simulink model "TVModel_Simulation"  (R2022a)
settings: Solver=FixedStepDiscrete  StartTime=0.0  StopTime=200  FixedStep=0.02  MaxStep=0.01  RelTol=1e-3
undefined symbols (not defined in the file or in its folder): TV
libraries: simulink x5, simulink_extras x3, dspstat3 x2, sharedTrackingLibrary x1, slpidlib x1, eeGeneralControl x1
(part 4 of 4)

== matlab function TVModel_Simulation/Subsystem/Subsystem1/Torque Distribution/MPC/ States/Extended Kalman Filter/state_update_kalman_simulink/f(x,u) ==
  data: x input; u input; xout output
function xout = state_update_kalman_simulink(x,u)

%% ~~~~~~~~~~~~~~~~~~~~~~~~~~~~~ Intro ~~~~~~~~~~~~~~~~~~~~~~~~~~~~~~~~~~~~
dt = 1/50;
%% ~~~~~~~~~~~~~~~~~~~~~~~~ Car parameters ~~~~~~~~~~~~~~~~~~~~~~~~~~~~~~~~
xout = zeros(3,1);
% ~~~~~~~~~~~~~~~~~~~~~~~~ General Parameters ~~~~~~~~~~~~~~~~~~~~~~~~~~~~~
g   = 9.81;            % [m/s^2]                          
wd  = 0.5;             % [~]         
wb  = 1.53;            % [~]          
tf  = 1.27;            % [m]          
tr  = 1.27;            % [m]          
m   = 195+75;          % [Kg]            
Iz  = 120;             % [Kg*m^2]         
a   = wb*wd;           % [m]            
b   = wb - a;          % [m]            
hcog = 0.29;           % [m]           
Fzf  = m*g/2*(wd);     % [N]                 
Fzr  = m*g/2*(1-wd);   % [N]                   
tau = 13.5;            % [~]          
rs  = 0.235;           % [m]           

% ~~~~~~~~~~~~~~~~~~~~~~~~~~~ Aero parameters ~~~~~~~~~~~~~~~~~~~~~~~~~~~~~
wbaero = 0.5542;       % [~]           
hcop = 0.576;          % [m]      
rho = 1.225;           % [Kg/m^3]     
CdA = 1.708;           % [m]     
ClA = 5.14;            % [m]    

% ~~~~~~~~~~~~~~~~~~~~~~~~~~ Other parameters ~~~~~~~~~~~~~~~~~~~~~~~~~~~~~

% ~~~~~~~~~~~~~~~~~~~~~~~~~~~ Set up states  ~~~~~~~~~~~~~~~~~~~~~~~~~~~~~~
vx = x(1);
vy = x(2);
r  = x(3);

% ~~~~~~~~~~~~~~~~~~~~~~~~~~~ Set up parameters ~~~~~~~~~~~~~~~~~~~~~~~~~~~
% delta    = u(1);
% kappa_FL = u(2);
% kappa_FR = u(3);
% kappa_RL = u(4);
% kappa_RR = u(5);
% Tbrk_FL  = u(6);
% Tbrk_FR  = u(7);
% Tbrk_RL  = u(8);
% Tbrk_RR  = u(9);
% ay       = u(10);
% ax       = u(11);
% T_FL     = u(12);
% T_FR     = u(13);
% T_RL     = u(14);
% T_RR     = u(15);

delta    = u(1);
kappa_FL = u(2);
kappa_FR = u(3);
kappa_RL = u(4);
kappa_RR = u(5);
T_FL     = u(6);
T_FR     = u(7);
T_RL     = u(8);
T_RR     = u(9);

ax = 0; ay = 0;
Tbrk_FL  = 0;
Tbrk_FR  = 0;
Tbrk_RL  = 0;
Tbrk_RR  = 0;
%% ~~~~~~~~~~~~~~~~~~~~~~~~~~ System Dynamics ~~~~~~~~~~~~~~~~~~~~~~~~~~~~~~

% ~~~~~~~~~~~~~~~~~~~~~~~~~~~ Aerodynamics ~~~~~~~~~~~~~~~~~~~~~~~~~~~~~~~~
Faerox = 0.5*rho*CdA*vx^2;
Faeroz = 0.5*rho*ClA*vx^2;

% ~~~~~~~~~~~~~~~~~~~~~~~~~~~ Slip Angles ~~~~~~~~~~~~~~~~~~~~~~~~~~~~~~~~~
alpha_FL =  (((vy + r*a)./(vx - r*tf/2)) - delta);
alpha_FR =  (((vy + r*a)./(vx + r*tf/2)) - delta);
alpha_RL =  (((vy - r*b)./(vx - r*tr/2)));     
alpha_RR =  (((vy - r*b)./(vx + r*tr/2)));     

% ~~~~~~~~~~~~~~~~~~~~~~~~~~~ Vertical loads ~~~~~~~~~~~~~~~~~~~~~~~~~~~~~~
Fz_FL = Fzf - 0.5*(m/tf*hcog).*ay + 0.5*Faeroz*wbaero - 0.5*Faerox/wb*hcop - 0.5*(m/wb*hcog).*ax;
Fz_FR = Fzf + 0.5*(m/tf*hcog).*ay + 0.5*Faeroz*wbaero - 0.5*Faerox/wb*hcop - 0.5*(m/wb*hcog).*ax;
Fz_RL = Fzr - 0.5*(m/tr*hcog).*ay + 0.5*Faeroz*(1-wbaero) + 0.5*Faerox/wb*hcop + 0.5*(m/wb*hcog).*ax;
Fz_RR = Fzr + 0.5*(m/tr*hcog).*ay + 0.5*Faeroz*(1-wbaero) + 0.5*Faerox/wb*hcop + 0.5*(m/wb*hcog).*ax;

% ~~~~~~~~~~~~~~~~~~~~~~~~~~ Lateral forces ~~~~~~~~~~~~~~~~~~~~~~~~~~~~~~~
muY = 1.5;
Fy_FL = (cos(0.95064*atan((41.4696*(kappa_FL - 0.00000078224999999999995925481499625675*Fz_FL + 0.00056678999999999995877686398415563))/((13.456699999999999661781657778192*alpha_FL - 0.51027806399999998717476046294905)^2 + 1.0)^(1/2) + (0.0012906*Fz_FL - 2.3215)*(atan((41.4696*(kappa_FL - 0.00000078224999999999995925481499625675*Fz_FL + 0.00056678999999999995877686398415563))/((13.456699999999999661781657778192*alpha_FL - 0.51027806399999998717476046294905)^2 + 1.0)^(1/2)) - (41.4696*(kappa_FL - 0.00000078224999999999995925481499625675*Fz_FL + 0.00056678999999999995877686398415563))/((13.456699999999999661781657778192*alpha_FL - 0.51027806399999998717476046294905)^2 + 1.0)^(1/2))))*(0.93*Fz_FL*(0.000071017999999999997795541162304289*Fz_FL - 0.14887799999999999779554116230429) - 0.93*Fz_FL*(0.00074656*Fz_FL + 0.37814) + Fz_FL*muY*sin(1.1962*atan((28888.097815192522084544179961085*sin(2.0*atan(0.00077863498204218704389788477193347*Fz_FL))*(0.000001140900000000000030428437547414*Fz_FL - 1.0*alpha_FL + (0.93*Fz_FL*(0.00074656*Fz_FL + 0.37814) + 1.1538900000000000822808488010196*Fz_FL*(0.00023917*Fz_FL - 1.57477))/(28888.097815192522084544179961085*sin(2.0*atan(0.00077863498204218704389788477193347*Fz_FL)) - 0.01) + 0.0023905000000000000467265115489113))/(1.1962*Fz_FL*muY + 0.01) - 1.0*(atan((28888.097815192522084544179961085*sin(2.0*atan(0.00077863498204218704389788477193347*Fz_FL))*(0.000001140900000000000030428437547414*Fz_FL - 1.0*alpha_FL + (0.93*Fz_FL*(0.00074656*Fz_FL + 0.37814) + 1.1538900000000000822808488010196*Fz_FL*(0.00023917*Fz_FL - 1.57477))/(28888.097815192522084544179961085*sin(2.0*atan(0.00077863498204218704389788477193347*Fz_FL)) - 0.01) + 0.0023905000000000000467265115489113))/(1.1962*Fz_FL*muY + 0.01)) - (28888.097815192522084544179961085*sin(2.0*atan(0.00077863498204218704389788477193347*Fz_FL))*(0.000001140900000000000030428437547414*Fz_FL - 1.0*alpha_FL + (0.93*Fz_FL*(0.00074656*Fz_FL + 0.37814) + 1.1538900000000000822808488010196*Fz_FL*(0.00023917*Fz_FL - 1.57477))/(28888.097815192522084544179961085*sin(2.0*atan(0.00077863498204218704389788477193347*Fz_FL)) - 0.01) + 0.0023905000000000000467265115489113))/(1.1962*Fz_FL*muY + 0.01))*(0.000039933999999999997276844965199416*Fz_FL - 0.52068399999999999727684496519942)*(0.47036*sign(0.000001140900000000000030428437547414*Fz_FL - 1.0*alpha_FL + (0.93*Fz_FL*(0.00074656*Fz_FL + 0.37814) + 1.1538900000000000822808488010196*Fz_FL*(0.00023917*Fz_FL - 1.57477))/(28888.097815192522084544179961085*sin(2.0*atan(0.00077863498204218704389788477193347*Fz_FL)) - 0.01) + 0.0023905000000000000467265115489113) - 7.9286)))))/cos(0.95064*atan((41.4696*(0.00000078224999999999995925481499625675*Fz_FL - 0.00056678999999999995877686398415563))/((13.456699999999999661781657778192*alpha_FL - 0.51027806399999998717476046294905)^2 + 1.0)^(1/2) + (0.0012906*Fz_FL - 2.3215)*(atan((41.4696*(0.00000078224999999999995925481499625675*Fz_FL - 0.00056678999999999995877686398415563))/((13.456699999999999661781657778192*alpha_FL - 0.51027806399999998717476046294905)^2 + 1.0)^(1/2)) - (41.4696*(0.00000078224999999999995925481499625675*Fz_FL - 0.00056678999999999995877686398415563))/((13.456699999999999661781657778192*alpha_FL - 0.51027806399999998717476046294905)^2 + 1.0)^(1/2)))) - (1.0*Fz_FL*muY*sin(1.9085*atan(16.5046*kappa_FL))*(0.0000027179999999999999299449271461526*Fz_FL - 1.1553830000000000000737188088351))/(225.17103248999997449603881705116*alpha_FL^2 + 1.0)^(1/2) + 400;
Fy_FR = (cos(0.95064*atan((41.4696*(kappa_FR - 0.00000078224999999999995925481499625675*Fz_FR + 0.00056678999999999995877686398415563))/((13.456699999999999661781657778192*alpha_FR - 0.51027806399999998717476046294905)^2 + 1.0)^(1/2) + (0.0012906*Fz_FR - 2.3215)*(atan((41.4696*(kappa_FR - 0.00000078224999999999995925481499625675*Fz_FR + 0.00056678999999999995877686398415563))/((13.456699999999999661781657778192*alpha_FR - 0.51027806399999998717476046294905)^2 + 1.0)^(1/2)) - (41.4696*(kappa_FR - 0.00000078224999999999995925481499625675*Fz_FR + 0.00056678999999999995877686398415563))/((13.456699999999999661781657778192*alpha_FR - 0.51027806399999998717476046294905)^2 + 1.0)^(1/2))))*(0.93*Fz_FR*(0.000071017999999999997795541162304289*Fz_FR - 0.14887799999999999779554116230429) - 0.93*Fz_FR*(0.00074656*Fz_FR + 0.37814) + Fz_FR*muY*sin(1.1962*atan((28888.097815192522084544179961085*sin(2.0*atan(0.00077863498204218704389788477193347*Fz_FR))*(0.000001140900000000000030428437547414*Fz_FR - 1.0*alpha_FR + (0.93*Fz_FR*(0.00074656*Fz_FR + 0.37814) + 1.1538900000000000822808488010196*Fz_FR*(0.00023917*Fz_FR - 1.57477))/(28888.097815192522084544179961085*sin(2.0*atan(0.00077863498204218704389788477193347*Fz_FR)) - 0.01) + 0.0023905000000000000467265115489113))/(1.1962*Fz_FR*muY + 0.01) - 1.0*(atan((28888.097815192522084544179961085*sin(2.0*atan(0.00077863498204218704389788477193347*Fz_FR))*(0.000001140900000000000030428437547414*Fz_FR - 1.0*alpha_FR + (0.93*Fz_FR*(0.00074656*Fz_FR + 0.37814) + 1.1538900000000000822808488010196*Fz_FR*(0.00023917*Fz_FR - 1.57477))/(28888.097815192522084544179961085*sin(2.0*atan(0.00077863498204218704389788477193347*Fz_FR)) - 0.01) + 0.0023905000000000000467265115489113))/(1.1962*Fz_FR*muY + 0.01)) - (28888.097815192522084544179961085*sin(2.0*atan(0.00077863498204218704389788477193347*Fz_FR))*(0.000001140900000000000030428437547414*Fz_FR - 1.0*alpha_FR + (0.93*Fz_FR*(0.00074656*Fz_FR + 0.37814) + 1.1538900000000000822808488010196*Fz_FR*(0.00023917*Fz_FR - 1.57477))/(28888.097815192522084544179961085*sin(2.0*atan(0.00077863498204218704389788477193347*Fz_FR)) - 0.01) + 0.0023905000000000000467265115489113))/(1.1962*Fz_FR*muY + 0.01))*(0.000039933999999999997276844965199416*Fz_FR - 0.52068399999999999727684496519942)*(0.47036*sign(0.000001140900000000000030428437547414*Fz_FR - 1.0*alpha_FR + (0.93*Fz_FR*(0.00074656*Fz_FR + 0.37814) + 1.1538900000000000822808488010196*Fz_FR*(0.00023917*Fz_FR - 1.57477))/(28888.097815192522084544179961085*sin(2.0*atan(0.00077863498204218704389788477193347*Fz_FR)) - 0.01) + 0.0023905000000000000467265115489113) - 7.9286)))))/cos(0.95064*atan((41.4696*(0.00000078224999999999995925481499625675*Fz_FR - 0.00056678999999999995877686398415563))/((13.456699999999999661781657778192*alpha_FR - 0.51027806399999998717476046294905)^2 + 1.0)^(1/2) + (0.0012906*Fz_FR - 2.3215)*(atan((41.4696*(0.00000078224999999999995925481499625675*Fz_FR - 0.00056678999999999995877686398415563))/((13.456699999999999661781657778192*alpha_FR - 0.51027806399999998717476046294905)^2 + 1.0)^(1/2)) - (41.4696*(0.00000078224999999999995925481499625675*Fz_FR - 0.00056678999999999995877686398415563))/((13.456699999999999661781657778192*alpha_FR - 0.51027806399999998717476046294905)^2 + 1.0)^(1/2)))) - (1.0*Fz_FR*muY*sin(1.9085*atan(16.5046*kappa_FR))*(0.0000027179999999999999299449271461526*Fz_FR - 1.1553830000000000000737188088351))/(225.17103248999997449603881705116*alpha_FR^2 + 1.0)^(1/2) + 400;
Fy_RL = (cos(0.95064*atan((41.4696*(kappa_RL - 0.00000078224999999999995925481499625675*Fz_RL + 0.00056678999999999995877686398415563))/((13.456699999999999661781657778192*alpha_RL - 0.51027806399999998717476046294905)^2 + 1.0)^(1/2) + (0.0012906*Fz_RL - 2.3215)*(atan((41.4696*(kappa_RL - 0.00000078224999999999995925481499625675*Fz_RL + 0.00056678999999999995877686398415563))/((13.456699999999999661781657778192*alpha_RL - 0.51027806399999998717476046294905)^2 + 1.0)^(1/2)) - (41.4696*(kappa_RL - 0.00000078224999999999995925481499625675*Fz_RL + 0.00056678999999999995877686398415563))/((13.456699999999999661781657778192*alpha_RL - 0.51027806399999998717476046294905)^2 + 1.0)^(1/2))))*(0.93*Fz_RL*(0.000071017999999999997795541162304289*Fz_RL - 0.14887799999999999779554116230429) - 0.93*Fz_RL*(0.00074656*Fz_RL + 0.37814) + Fz_RL*muY*sin(1.1962*atan((28888.097815192522084544179961085*sin(2.0*atan(0.00077863498204218704389788477193347*Fz_RL))*(0.000001140900000000000030428437547414*Fz_RL - 1.0*alpha_RL + (0.93*Fz_RL*(0.00074656*Fz_RL + 0.37814) + 1.1538900000000000822808488010196*Fz_RL*(0.00023917*Fz_RL - 1.57477))/(28888.097815192522084544179961085*sin(2.0*atan(0.00077863498204218704389788477193347*Fz_RL)) - 0.01) + 0.0023905000000000000467265115489113))/(1.1962*Fz_RL*muY + 0.01) - 1.0*(atan((28888.097815192522084544179961085*sin(2.0*atan(0.00077863498204218704389788477193347*Fz_RL))*(0.000001140900000000000030428437547414*Fz_RL - 1.0*alpha_RL + (0.93*Fz_RL*(0.00074656*Fz_RL + 0.37814) + 1.1538900000000000822808488010196*Fz_RL*(0.00023917*Fz_RL - 1.57477))/(28888.097815192522084544179961085*sin(2.0*atan(0.00077863498204218704389788477193347*Fz_RL)) - 0.01) + 0.0023905000000000000467265115489113))/(1.1962*Fz_RL*muY + 0.01)) - (28888.097815192522084544179961085*sin(2.0*atan(0.00077863498204218704389788477193347*Fz_RL))*(0.000001140900000000000030428437547414*Fz_RL - 1.0*alpha_RL + (0.93*Fz_RL*(0.00074656*Fz_RL + 0.37814) + 1.1538900000000000822808488010196*Fz_RL*(0.00023917*Fz_RL - 1.57477))/(28888.097815192522084544179961085*sin(2.0*atan(0.00077863498204218704389788477193347*Fz_RL)) - 0.01) + 0.0023905000000000000467265115489113))/(1.1962*Fz_RL*muY + 0.01))*(0.000039933999999999997276844965199416*Fz_RL - 0.52068399999999999727684496519942)*(0.47036*sign(0.000001140900000000000030428437547414*Fz_RL - 1.0*alpha_RL + (0.93*Fz_RL*(0.00074656*Fz_RL + 0.37814) + 1.1538900000000000822808488010196*Fz_RL*(0.00023917*Fz_RL - 1.57477))/(28888.097815192522084544179961085*sin(2.0*atan(0.00077863498204218704389788477193347*Fz_RL)) - 0.01) + 0.0023905000000000000467265115489113) - 7.9286)))))/cos(0.95064*atan((41.4696*(0.00000078224999999999995925481499625675*Fz_RL - 0.00056678999999999995877686398415563))/((13.456699999999999661781657778192*alpha_RL - 0.51027806399999998717476046294905)^2 + 1.0)^(1/2) + (0.0012906*Fz_RL - 2.3215)*(atan((41.4696*(0.00000078224999999999995925481499625675*Fz_RL - 0.00056678999999999995877686398415563))/((13.456699999999999661781657778192*alpha_RL - 0.51027806399999998717476046294905)^2 + 1.0)^(1/2)) - (41.4696*(0.00000078224999999999995925481499625675*Fz_RL - 0.00056678999999999995877686398415563))/((13.456699999999999661781657778192*alpha_RL - 0.51027806399999998717476046294905)^2 + 1.0)^(1/2)))) - (1.0*Fz_RL*muY*sin(1.9085*atan(16.5046*kappa_RL))*(0.0000027179999999999999299449271461526*Fz_RL - 1.1553830000000000000737188088351))/(225.17103248999997449603881705116*alpha_RL^2 + 1.0)^(1/2) + 400;
Fy_RR = (cos(0.95064*atan((41.4696*(kappa_RR - 0.00000078224999999999995925481499625675*Fz_RR + 0.00056678999999999995877686398415563))/((13.456699999999999661781657778192*alpha_RR - 0.51027806399999998717476046294905)^2 + 1.0)^(1/2) + (0.0012906*Fz_RR - 2.3215)*(atan((41.4696*(kappa_RR - 0.00000078224999999999995925481499625675*Fz_RR + 0.00056678999999999995877686398415563))/((13.456699999999999661781657778192*alpha_RR - 0.51027806399999998717476046294905)^2 + 1.0)^(1/2)) - (41.4696*(kappa_RR - 0.00000078224999999999995925481499625675*Fz_RR + 0.00056678999999999995877686398415563))/((13.456699999999999661781657778192*alpha_RR - 0.51027806399999998717476046294905)^2 + 1.0)^(1/2))))*(0.93*Fz_RR*(0.000071017999999999997795541162304289*Fz_RR - 0.14887799999999999779554116230429) - 0.93*Fz_RR*(0.00074656*Fz_RR + 0.37814) + Fz_RR*muY*sin(1.1962*atan((28888.097815192522084544179961085*sin(2.0*atan(0.00077863498204218704389788477193347*Fz_RR))*(0.000001140900000000000030428437547414*Fz_RR - 1.0*alpha_RR + (0.93*Fz_RR*(0.00074656*Fz_RR + 0.37814) + 1.1538900000000000822808488010196*Fz_RR*(0.00023917*Fz_RR - 1.57477))/(28888.097815192522084544179961085*sin(2.0*atan(0.00077863498204218704389788477193347*Fz_RR)) - 0.01) + 0.0023905000000000000467265115489113))/(1.1962*Fz_RR*muY + 0.01) - 1.0*(atan((28888.097815192522084544179961085*sin(2.0*atan(0.00077863498204218704389788477193347*Fz_RR))*(0.000001140900000000000030428437547414*Fz_RR - 1.0*alpha_RR + (0.93*Fz_RR*(0.00074656*Fz_RR + 0.37814) + 1.1538900000000000822808488010196*Fz_RR*(0.00023917*Fz_RR - 1.57477))/(28888.097815192522084544179961085*sin(2.0*atan(0.00077863498204218704389788477193347*Fz_RR)) - 0.01) + 0.0023905000000000000467265115489113))/(1.1962*Fz_RR*muY + 0.01)) - (28888.097815192522084544179961085*sin(2.0*atan(0.00077863498204218704389788477193347*Fz_RR))*(0.000001140900000000000030428437547414*Fz_RR - 1.0*alpha_RR + (0.93*Fz_RR*(0.00074656*Fz_RR + 0.37814) + 1.1538900000000000822808488010196*Fz_RR*(0.00023917*Fz_RR - 1.57477))/(28888.097815192522084544179961085*sin(2.0*atan(0.00077863498204218704389788477193347*Fz_RR)) - 0.01) + 0.0023905000000000000467265115489113))/(1.1962*Fz_RR*muY + 0.01))*(0.000039933999999999997276844965199416*Fz_RR - 0.52068399999999999727684496519942)*(0.47036*sign(0.000001140900000000000030428437547414*Fz_RR - 1.0*alpha_RR + (0.93*Fz_RR*(0.00074656*Fz_RR + 0.37814) + 1.1538900000000000822808488010196*Fz_RR*(0.00023917*Fz_RR - 1.57477))/(28888.097815192522084544179961085*sin(2.0*atan(0.00077863498204218704389788477193347*Fz_RR)) - 0.01) + 0.0023905000000000000467265115489113) - 7.9286)))))/cos(0.95064*atan((41.4696*(0.00000078224999999999995925481499625675*Fz_RR - 0.00056678999999999995877686398415563))/((13.456699999999999661781657778192*alpha_RR - 0.51027806399999998717476046294905)^2 + 1.0)^(1/2) + (0.0012906*Fz_RR - 2.3215)*(atan((41.4696*(0.00000078224999999999995925481499625675*Fz_RR - 0.00056678999999999995877686398415563))/((13.456699999999999661781657778192*alpha_RR - 0.51027806399999998717476046294905)^2 + 1.0)^(1/2)) - (41.4696*(0.00000078224999999999995925481499625675*Fz_RR - 0.00056678999999999995877686398415563))/((13.456699999999999661781657778192*alpha_RR - 0.51027806399999998717476046294905)^2 + 1.0)^(1/2)))) - (1.0*Fz_RR*muY*sin(1.9085*atan(16.5046*kappa_RR))*(0.0000027179999999999999299449271461526*Fz_RR - 1.1553830000000000000737188088351))/(225.17103248999997449603881705116*alpha_RR^2 + 1.0)^(1/2) + 400;

% ~~~~~~~~~~~~~~~~~~~~~~~~~~ Longitudinal forces ~~~~~~~~~~~~~~~~~~~~~~~~~~
Fx_FL = (T_FL.*tau - Tbrk_FL)/rs;
Fx_FR = (T_FR.*tau - Tbrk_FR)/rs;
Fx_RL = (T_RL.*tau - Tbrk_RL)/rs;
Fx_RR = (T_RR.*tau - Tbrk_RR)/rs;

% ~~~~~~~~~~~~~~~~~~~~~~~~~~~ E.o.M. Balance ~~~~~~~~~~~~~~~~~~~~~~~~~~~~~~
X1 = (Fx_FL + Fx_FR).*cos(delta) - (Fy_FL + Fy_FR).*sin(delta);
X2 = Fx_RL + Fx_RR;
deltaX1 = ((Fx_FR - Fx_FL).*cos(delta) - (Fy_FR - Fy_FL).*sin(delta))/2;
deltaX2 = (Fx_RR - Fx_RL)/2;

Y1 = (Fy_FL + Fy_FR).*cos(delta) + (Fx_FL + Fx_FR).*sin(delta);
Y2 = Fy_RL + Fy_RR;

X = X1 + X2 - Faerox;
Y = Y1 + Y2;
N = Y1*a - Y2*b + deltaX1*tf + deltaX2*tr;

% ~~~~~~~~~~~~~~~~~~~~~~~~~~~ System Dynamics f(x,u) ~~~~~~~~~~~~~~~~~~~~~~
xout(1) =  1/m.*(X + vy.*r)*dt + x(1);
xout(2) =  1/m.*(Y - vx.*r)*dt + x(2);
xout(3) =  1/Iz.*(N)*dt + x(3);
end

== matlab function TVModel_Simulation/Subsystem/Subsystem1/Torque Distribution/MPC/ States/Yrd 0 When Steering 0/Linear Activation ==
  data: in_1 input; epsilon input; out output; in_2 input
function out = fcn(in_1,epsilon,in_2)

out = in_1*epsilon + in_2*(1 - epsilon) ;

== matlab function TVModel_Simulation/Subsystem/Subsystem1/Torque Distribution/MPC/Faults detection/Subsystem/MATLAB Function ==
  data: T input; Tnew output; Plim input; Eta input; Omega input; Torque input; Omega_motors input; k output; fx output; brake_flag input
function [Tnew,k,fx] = fcn(T,Plim,Eta,Omega,Torque,Omega_motors,brake_flag)

Tnew = zeros(4,1);
fx = 10^3;
k      = 0;

exit   = 0;
dT     = 0;
eps    = 0.01;
h      = 0.3;
dT_new = 0;

eta_Plim = 1;

while exit == 0

    if brake_flag == 0;
        Tnew(1) = T(1) - dT;
        Tnew(2) = T(2) - dT;
        Tnew(3) = T(3) - dT;
        Tnew(4) = T(4) - dT;  
    
        eta = efficiency(Eta,Omega,Torque,Tnew,Omega_motors);
   

        for i = 1 : 4
            if Tnew(i) <= 0 
               Tnew(i) = 0;
            end
        end
    else
        Tnew(1) = T(1) + dT;
        Tnew(2) = T(2) + dT;
        Tnew(3) = T(3) + dT;
        Tnew(4) = T(4) + dT;  
    
        eta = efficiency(Eta,Omega,Torque,Tnew,Omega_motors);
   

        for i = 1 : 4
            if Tnew(i) >= 0 
               Tnew(i) = 0;
            end
        end
    end
%     eta1_hplus = efficiency(Eta,Omega,Torque,T1 - (dT + h),w1);
%     eta1_hminus = efficiency(Eta,Omega,Torque,T1 - (dT -h),w1);
%     eta2_hplus = efficiency(Eta,Omega,Torque,T2 - (dT + h),w2);
%     eta2_hminus = efficiency(Eta,Omega,Torque,T2 - (dT -h),w2);  
    fx = ( dot(Tnew./eta,Omega_motors') - Plim*eta_Plim );
    dT_new = dT + h;
    
%     fdotx = (-1/eta1/ ((eta1_hplus - eta1_hminus)/(2*h)) -1/eta2/ ((eta2_hplus - eta2_hminus)/(2*h)) );
%     dT_new = dT -  fx/fdotx;
    if k >= 100 || fx<0 || isnan(fx)
       exit = 1;
    else 
       dT = dT_new;
       k = k + 1;
    end

end

end

function eta = efficiency(Eta,Omega,Torque,T,w)    
         eta = interp2(Torque,Omega,Eta,abs(T),abs(w),"linear");
end

== matlab function TVModel_Simulation/Subsystem/Subsystem1/Torque Distribution/MPC/Polytropic Matrix/MATLAB Function ==
  data: y output; Limit input
function y = fcn(Limit)

% Limit = [1;1;1;1];

% C = [0 , 0 , 0 , 1 , 1 , 1 , 1;
%      0 , 0 , 0 , Limit(1) , Limit(2) , Limit(3) , Limit(4);
%      0 , 0 , 0 , 0 , 1 , 0 ,-1;
%      0 , 0 , 0 , 1 , 0 ,-1 , 0];
% 
% y = C(:);

y = [0,0,0,0,0,0,0,0,0,0,0,0,1,Limit(1),0,1,1,Limit(2),1,0,1,Limit(3),0,-1,1,Limit(4),-1,0]';

== matlab function TVModel_Simulation/Subsystem/Subsystem1/Torque Distribution/MPC/States constraints/Cross Check ==
  data: ubu input; param input; ubu output; lbu input; lbu output
function [ubu,lbu] = fcn(ubu,param,lbu)
flag = param(1);
ubu_target = param(2:5);
lbu_target = param(6:9);
lbu_max = param(10);
switch flag
    case 0 %% Check cross between bounds
        for i = 1 : 4
            if lbu(i) > ubu(i)
               lbu(i) = ubu(i) - lbu_max;
            end
        end
    case 1 %% Check for low YRD Accelerating
        for i = 1 :4
            ubu(i) = ubu_target(i);
            lbu(i) = 0;
        end
    case 2 %% Check for low YRD Braking
        for i = 1:4
            lbu(i) = lbu_target(i);
            ubu(i) = 0;
        end
    case 3 %% Overlapping
        for i = 1:4
            lbu(i) = 0;
            ubu(i) = 0;
        end
end

== matlab function TVModel_Simulation/Subsystem/Subsystem1/Torque Distribution/MPC/Weights generation/Efficiency limit/MATLAB Function ==
  data: u input; u output; T input
function u = fcn(u,T)

for i = 1 : 4
    if T(i) <= 0 
       u(i) = 0; 
    end
end

== matlab function TVModel_Simulation/Subsystem/Subsystem1/Torque Distribution/MPC/Weights generation/MATLAB Function ==
  data: u input; y output
function y = fcn(u)

Q = diag([u(1),u(2),u(3),u(4),u(5),u(6),u(7)]);
R = diag([u(8),u(9),u(10),u(11)]);
unscale = 50;
W = unscale * blkdiag(Q, R);
y = W(:);

== matlab function TVModel_Simulation/Subsystem/Subsystem1/Torque Distribution/MPC/Weights generation/Non-Linear Activation ==
  data: in_1 input; epsilon input; out output; in_2 input
function out = fcn(in_1,epsilon,in_2)

beta = 4;
epsilon = 1/(1 + (epsilon/(1-epsilon))^(-beta) );

out = in_1*epsilon + in_2*(1 - epsilon) ;

== matlab function TVModel_Simulation/Subsystem/Subsystem1/Torque Distribution/Reference Tracking/MATLAB Function ==
  data: LUT_brk input; brk input; YRD output; LUT_thr input
function YRD = fcn(LUT_brk,brk,LUT_thr)

YRD = LUT_brk*brk + LUT_thr*(1 - brk) ;

== stateflow chart TVModel_Simulation/Subsystem/Subsystem1/Torque Limits/Torque Request/T_Req_Chart ==
  state Brake
    en:
    t_req=1;
  state Throttle
    en:
    t_req=0;
  (default) -> Throttle
  Brake -> Throttle : [brake<=0 && throttle<0.05]
  Throttle -> Brake : [brake>0]
  data: brake input; throttle input; t_req output

== matlab function TVModel_Simulation/Subsystem/Subsystem1/Slip Control/Traction_PID/TC ==
  data: slip_ratio_target input; slip_ratio input; t_pid output; kp input; ki input; time_step input
function t_pid = fcn(slip_ratio_target, slip_ratio, kp, ki, time_step)

%memory allocation
t_pid         = zeros(1, 4);
slip_error    = zeros(1, 4);

%slip errors
slip_error(1) = slip_ratio_target - slip_ratio(1);
slip_error(2) = slip_ratio_target - slip_ratio(2);
slip_error(3) = slip_ratio_target - slip_ratio(3);
slip_error(4) = slip_ratio_target - slip_ratio(4);

%% FL
    t_pid(1) = slip_error(1)*kp + trapz(slip_error(1)*ki);
%% FR
    t_pid(2) = slip_error(2)*kp + trapz(slip_error(2)*ki);
%% RL
    t_pid(3) = slip_error(3)*kp + trapz(slip_error(3)*ki);
%% RR
    t_pid(4) = slip_error(4)*kp + trapz(slip_error(4)*ki);

== stateflow chart TVModel_Simulation/Subsystem/Subsystem1/Slip Control/Traction_PID/TC_Activation_Logic ==
  state TS_ON
    state TC_OFF
      en,du:
      t_max_pid(1:4) = t_limit_positive(1:4);
    state TC_ON
      state FL [parallel]
        settings: executionOrder=1
        state TC_INACTIVE
          en:
          t_max_pid(1) = t_limit_positive(1);
          du:
          t_max_pid(1) = t_limit_positive(1);
        state TC_ACTIVE
          en:
          t_max_pid(1) = abs(t_actual(1));
          du:
          t_max_pid(1) = t_max_pid(1)+t_pid(1);
        (default) -> TS_ON.TC_ON.FL.TC_INACTIVE
        TS_ON.TC_ON.FL.TC_INACTIVE -> TS_ON.TC_ON.FL.TC_ACTIVE : [slip_ratio(1) >= slip_ratio_target]
        TS_ON.TC_ON.FL.TC_ACTIVE -> TS_ON.TC_ON.FL.TC_INACTIVE : [slip_ratio(1) < slip_ratio_target*0.3]
      state FR [parallel]
        settings: executionOrder=2
        state TC_ACTIVE
          en:
          t_max_pid(2) = abs(t_actual(2));
          du:
          t_max_pid(2) = t_max_pid(2)+t_pid(2);
        state TC_INACTIVE
          en:
          t_max_pid(2) = t_limit_positive(2);
          du:
          t_max_pid(2) = t_limit_positive(2);
        (default) -> TS_ON.TC_ON.FR.TC_INACTIVE
        TS_ON.TC_ON.FR.TC_INACTIVE -> TS_ON.TC_ON.FR.TC_ACTIVE : [slip_ratio(2) >= slip_ratio_target]
        TS_ON.TC_ON.FR.TC_ACTIVE -> TS_ON.TC_ON.FR.TC_INACTIVE : [slip_ratio(2) < slip_ratio_target*0.3]
      state RL [parallel]
        settings: executionOrder=3
        state TC_INACTIVE
          en:
          t_max_pid(3) = t_limit_positive(3);
          du:
          t_max_pid(3) = t_limit_positive(3);
        state TC_ACTIVE
          en:
          t_max_pid(3) = abs(t_actual(3));
          du:
          t_max_pid(3) = t_max_pid(3)+t_pid(3);
        (default) -> TS_ON.TC_ON.RL.TC_INACTIVE
        TS_ON.TC_ON.RL.TC_INACTIVE -> TS_ON.TC_ON.RL.TC_ACTIVE : [slip_ratio(3) >= slip_ratio_target]
        TS_ON.TC_ON.RL.TC_ACTIVE -> TS_ON.TC_ON.RL.TC_INACTIVE : [slip_ratio(3) < slip_ratio_target*0.3]
      state RR [parallel]
        settings: executionOrder=4
        state TC_ACTIVE
          en:
          t_max_pid(4) = abs(t_actual(4));
          du:
          t_max_pid(4) = t_max_pid(4)+t_pid(4);
        state TC_INACTIVE
          en:
          t_max_pid(4) = t_limit_positive(4);
          du:
          t_max_pid(4) = t_limit_positive(4);
        (default) -> TS_ON.TC_ON.RR.TC_INACTIVE
        TS_ON.TC_ON.RR.TC_INACTIVE -> TS_ON.TC_ON.RR.TC_ACTIVE : [slip_ratio(4) >= slip_ratio_target]
        TS_ON.TC_ON.RR.TC_ACTIVE -> TS_ON.TC_ON.RR.TC_INACTIVE : [slip_ratio(4) < slip_ratio_target*0.3]
    (default) -> TC_OFF
    TC_ON -> TC_OFF : [tc_flag == 0]
    TC_OFF -> TC_ON : [tc_flag == 1]
  state TS_OFF
    en:
    t_max_pid(1:4) = zeros(4,1);
  (default) -> TS_OFF
  TS_OFF -> TS_ON : [rtd_flag == 1]
  TS_ON -> TS_OFF : [rtd_flag == 0]
  data: t_pid input; t_actual input; rtd_flag input; tc_flag input; t_max_pid output =zeros(4, 1); t_limit_positive input; slip_ratio input; slip_ratio_target input
